simulink model "practica11"  (R2024a)
settings: Solver=VariableStepAuto  StartTime=0.0  StopTime=10.0  RelTol=1e-3

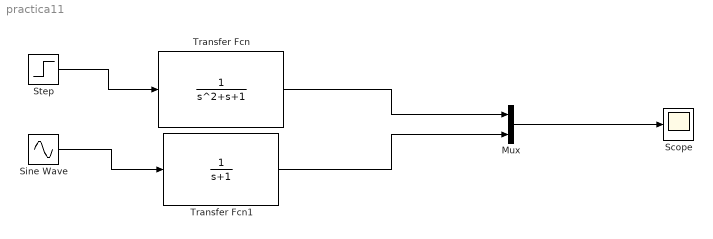
== system practica11 ==
  Mux : Mux  Inputs=2
  Scope : Scope
  Sine Wave : Sin  Frequency=60  SampleTime=0
  Step : Step  Time=0  SampleTime=0
  Transfer Fcn : TransferFcn  Denominator=[1 1 1 ]
  Transfer Fcn1 : TransferFcn  Denominator="[1 1  ]"
  wires:
  Sine Wave/1 -> Transfer Fcn1/1
  Step/1 -> Transfer Fcn/1
  Transfer Fcn1/1 -> Mux/2
  Transfer Fcn/1 -> Mux/1
  Mux/1 -> Scope/1
